simulink model "Inverted_Pendulum9"  (R2020b)
settings: Solver=ode1  StartTime=0.0  StopTime=5  FixedStep=T  RelTol=1e-3  EnableMultiTasking=on
model workspace (MAT data in the model file):
  Var = 0
values from neighbouring files (symbols this model uses):
  binb1 = reshape(psi(binLayerRanges(1, 3):binLayerRanges(1, 4)), binLayers(2), 1)    [main.m]
  binb2 = reshape(psi(binLayerRanges(2, 3):binLayerRanges(2, 4)), binLayers(3), 1)    [main.m]
  binb3 = reshape(psi(binLayerRanges(3, 3):binLayerRanges(3, 4)), binLayers(4), 1)    [main.m]
  binW1 = reshape(psi(binLayerRanges(1, 1):binLayerRanges(1, 2)), binLayers(2), binLayers(1))    [main.m]
  binW2 = reshape(psi(binLayerRanges(2, 1):binLayerRanges(2, 2)), binLayers(3), binLayers(2))    [main.m]
  binW3 = reshape(psi(binLayerRanges(3, 1):binLayerRanges(3, 2)), binLayers(4), binLayers(3))    [main.m]
  control1b1 = reshape(theta1(control1LayerRanges(1, 3):control1LayerRanges(1, 4)), control1Layers(2), 1)    [main.m]
  control1b2 = reshape(theta1(control1LayerRanges(2, 3):control1LayerRanges(2, 4)), control1Layers(3), 1)    [main.m]
  control1b3 = reshape(theta1(control1LayerRanges(3, 3):control1LayerRanges(3, 4)), control1Layers(4), 1)    [main.m]
  control1W1 = reshape(theta1(control1LayerRanges(1, 1):control1LayerRanges(1, 2)), control1Layers(2), control1Layers(1))    [main.m]
  control1W2 = reshape(theta1(control1LayerRanges(2, 1):control1LayerRanges(2, 2)), control1Layers(3), control1Layers(2))    [main.m]
  control1W3 = reshape(theta1(control1LayerRanges(3, 1):control1LayerRanges(3, 2)), control1Layers(4), control1Layers(3))    [main.m]
  control2b1 = reshape(theta2(control2LayerRanges(1, 3):control2LayerRanges(1, 4)), control2Layers(2), 1)    [main.m]
  control2b2 = reshape(theta2(control2LayerRanges(2, 3):control2LayerRanges(2, 4)), control2Layers(3), 1)    [main.m]
  control2b3 = reshape(theta2(control2LayerRanges(3, 3):control2LayerRanges(3, 4)), control2Layers(4), 1)    [main.m]
  control2W1 = reshape(theta2(control2LayerRanges(1, 1):control2LayerRanges(1, 2)), control2Layers(2), control2Layers(1))    [main.m]
  control2W2 = reshape(theta2(control2LayerRanges(2, 1):control2LayerRanges(2, 2)), control2Layers(3), control2Layers(2))    [main.m]
  control2W3 = reshape(theta2(control2LayerRanges(3, 1):control2LayerRanges(3, 2)), control2Layers(4), control2Layers(3))    [main.m]
  control3b1 = reshape(theta3(control3LayerRanges(1, 3):control3LayerRanges(1, 4)), control3Layers(2), 1)    [main.m]
  control3b2 = reshape(theta3(control3LayerRanges(2, 3):control3LayerRanges(2, 4)), control3Layers(3), 1)    [main.m]
  control3b3 = reshape(theta3(control3LayerRanges(3, 3):control3LayerRanges(3, 4)), control3Layers(4), 1)    [main.m]
  control3W1 = reshape(theta3(control3LayerRanges(1, 1):control3LayerRanges(1, 2)), control3Layers(2), control3Layers(1))    [main.m]
  control3W2 = reshape(theta3(control3LayerRanges(2, 1):control3LayerRanges(2, 2)), control3Layers(3), control3Layers(2))    [main.m]
  control3W3 = reshape(theta3(control3LayerRanges(3, 1):control3LayerRanges(3, 2)), control3Layers(4), control3Layers(3))    [main.m]
  g = 9.81    [Inverted_Pendulum9_data.m]
  Jp = m*Lp*Lp/3    (= 0.0056549032375)    [Inverted_Pendulum9_data.m]
  K1 = K(1,1)    [Inverted_Pendulum9_data.m]
  K2 = K(1,2)    [Inverted_Pendulum9_data.m]
  K3 = K(1,3)    [Inverted_Pendulum9_data.m]
  K4 = K(1,4)    [Inverted_Pendulum9_data.m]
  Kenc = 2.275e-5    (= 2.275e-05)    [Inverted_Pendulum9_data.m]    (also in cartpole_data.m = 2.27489350843e-05)
  Kt = 0.00767    [Inverted_Pendulum9_data.m]
  Lp = 0.6413/2    (= 0.32065)    [Inverted_Pendulum9_data.m]
  M = 0.57    [Inverted_Pendulum9_data.m]    (also in cartpole_data.m)
  m = 0.165    [Inverted_Pendulum9_data.m]
  Nenc = 4096    [Inverted_Pendulum9_data.m]    (also in cartpole_data.m)
  R = 2.6    [Inverted_Pendulum9_data.m]    (also in cartpole_data.m)
  rg = 3.71    [Inverted_Pendulum9_data.m]    (also in cartpole_data.m)
  rm = 6.35e-3    (= 0.00635)    [Inverted_Pendulum9_data.m]    (also in cartpole_data.m)
  T = 0.001    [Inverted_Pendulum9_data.m]    (also in cartpole_data.m)
  theta_0 = 1*pi/180    (= 0.0174532925199)    [Inverted_Pendulum9_data.m]
  Vmax = 10    [Inverted_Pendulum9_data.m]
  x_0 = 0*0.1    (= 0)    [Inverted_Pendulum9_data.m]
undefined symbols (not defined in the file or in its folder): af, bf, magnitude
libraries: simulink x1
settings Model: ExtModeArmWhenConnect=off  Creator=johnchiasson  LastModifiedBy=nardosashenafi
settings DataIOCC: LimitDataPoints=on  SaveFormat=Array  SignalLoggingSaveFormat=ModelDataLogs  ReturnWorkspaceOutputs=off
settings OptimizationCC: BooleanDataType=off  OptimizeBlockIOStorage=off  BufferReuse=off  GlobalBufferReuse=off  ExpressionFolding=off  ExpressionDepthLimit=2147483647  LocalBlockOutputs=off  LifeSpan=inf  OptimizeDataStoreBuffers=off  BusAssignmentInplaceUpdate=off
settings DebuggingCC: SaveWithParameterizedLinksMsg=none  UnderspecifiedInitializationDetection=Classic  MergeDetectMultiDrivingBlocksExec=none  SignalResolutionControl=TryResolveAllWithWarning  MultiTaskDSMMsg=warning  MultiTaskCondExecSysMsg=none  FcnCallInpInsideContextMsg=warning  StateNameClashWarn=warning  SFUnexpectedBacktrackingDiag=warning  SFNoUnconditionalDefaultTransitionDiag=warning  SFExecutionAtInitializationDiag=none  UnderSpecifiedDimensionMsg=warning  ArithmeticOperatorsInVariantConditions=warning
settings HardwareCC: ProdBitPerPointer=32  ProdBitPerSizeT=32  ProdBitPerPtrDiffT=32  ProdLargestAtomicFloat=None  ProdIntDivRoundTo=Undefined  ProdEndianess=Unspecified  ProdWordSize=32  ProdHWDeviceType=32-bit Generic  TargetUnknown=on
settings ModelReferenceCC: PropagateSignalLabelsOutOfModel=off
settings SFSimCC: SimUseLocalCustomCode=off  CustomCodeUndefinedFunction=UseInterfaceOnly
settings RTWCC: SystemTargetFile=wincon.tlc  MakeCommand=make_wc  TemplateMakefile=nt_msvc.tmf  RTWUseLocalCustomCode=off
settings CodeAppCC: StateflowObjectComments=on
settings STFCustomTargetCC: ModelReferenceCompliant=off  ConcurrentExecutionCompliant=off  MATLABClassNameForMDSCustomization=Simulink.SoftwareTarget.TargetSpecificTriggerConfigurationBase  CPPClassGenCompliant=off  SystemTargetFile=wincon.tlc
settings ConfigComp: CovMetricSettings=dw  CovSaveCumulativeToWorkspaceVar=on  CovSaveSingleToWorkspaceVar=on  CovExternalEMLEnable=off  CovSFcnEnable=off

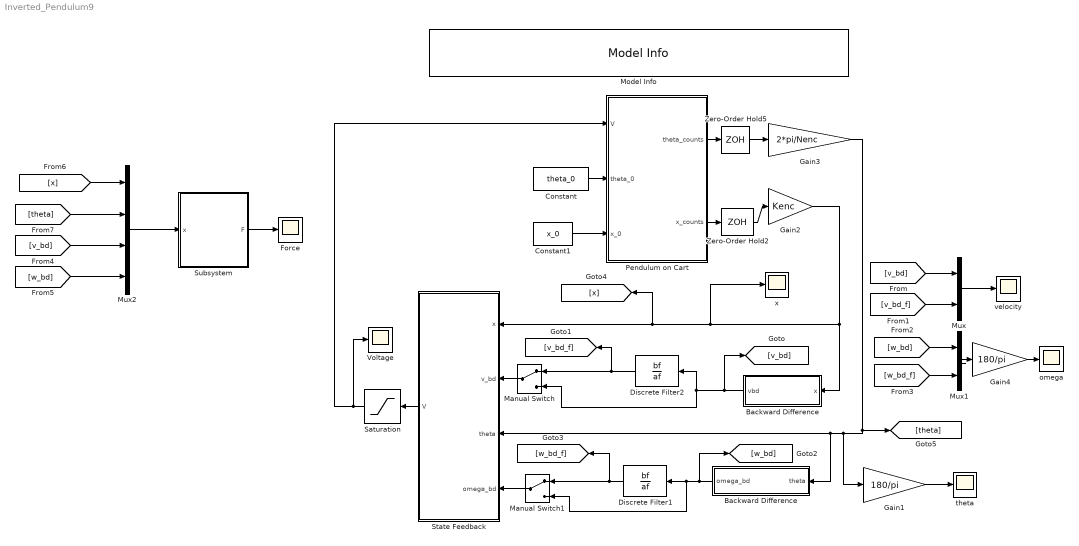
== system Inverted_Pendulum9 ==
  Backward Difference : Subsystem
  "Backward Difference " : Subsystem
  Constant : Constant  Value=theta_0
  Constant1 : Constant  Value=x_0
  Discrete Filter1 : DiscreteFilter  Numerator=bf  Denominator=af
  Discrete Filter2 : DiscreteFilter  Numerator=bf  Denominator=af
  Force : Scope
  Gain1 : Gain  Gain=180/pi  SaturateOnIntegerOverflow=on  OutDataTypeStr=Inherit: Same as input  ParamDataTypeStr=Inherit: Same as input
  Gain2 : Gain  Gain=Kenc  SaturateOnIntegerOverflow=on  OutDataTypeStr=Inherit: Same as input  ParamDataTypeStr=Inherit: Same as input
  Gain3 : Gain  Gain=2*pi/Nenc  SaturateOnIntegerOverflow=on  OutDataTypeStr=Inherit: Same as input  ParamDataTypeStr=Inherit: Same as input
  Gain4 : Gain  Gain=180/pi  SaturateOnIntegerOverflow=on  OutDataTypeStr=Inherit: Same as input  ParamDataTypeStr=Inherit: Same as input
  Manual Switch : ManualSwitch
  Manual Switch1 : ManualSwitch
  Model Info : simulink/Model-Wide Utilities/Model Info  Frame=on  DisplayStringWithTags=Inverted Pendulum on the Cart Model with Encoder Models  HorizontalTextAlignment=Center  LeftAlignmentValue=0.5
  Mux : Mux  Inputs=2
  Mux1 : Mux  Inputs=2
  Mux2 : Mux
  Pendulum on Cart : Subsystem
  Saturation : Saturate  UpperLimit=Vmax  LowerLimit=-Vmax
  State Feedback : Subsystem
  Subsystem : Subsystem
  Voltage : Scope
  Zero-Order Hold2 : ZeroOrderHold  SampleTime=T
  Zero-Order Hold5 : ZeroOrderHold  SampleTime=T
  omega : Scope
  theta : Scope
  velocity : Scope
  x : Scope
  wires:
  State Feedback/1(V) -> Saturation/1
  Constant/1 -> Pendulum on Cart/2(theta_0)
  Constant1/1 -> Pendulum on Cart/3(x_0)
  "Backward Difference "/1(vbd) -> Manual Switch/2, Discrete Filter2/1, [v_bd]
  Pendulum on Cart/2(x_counts) -> Zero-Order Hold2/1
  Pendulum on Cart/1(theta_counts) -> Zero-Order Hold5/1
  Saturation/1 -> Pendulum on Cart/1(V), Voltage/1
  Mux/1 -> velocity/1
  [v_bd] -> Mux/1
  [v_bd_f] -> Mux/2
  Backward Difference/1(omega_bd) -> [w_bd], Manual Switch1/2, Discrete Filter1/1
  Mux1/1 -> Gain4/1
  [w_bd] -> Mux1/1
  [w_bd_f] -> Mux1/2
  Gain1/1 -> theta/1
  Gain4/1 -> omega/1
  Gain3/1 -> Gain1/1, State Feedback/3(theta), Backward Difference/1(theta), [theta]
  Gain2/1 -> [x], State Feedback/1(x), x/1, "Backward Difference "/1(x)
  Zero-Order Hold5/1 -> Gain3/1
  Zero-Order Hold2/1 -> Gain2/1
  Discrete Filter2/1 -> Manual Switch/1, [v_bd_f]
  Discrete Filter1/1 -> [w_bd_f], Manual Switch1/1
  Manual Switch/1 -> State Feedback/2(v_bd)
  Manual Switch1/1 -> State Feedback/4(omega_bd)
  [w_bd] -> Mux2/4
  [v_bd] -> Mux2/3
  [theta] -> Mux2/2
  [x] -> Mux2/1
  Mux2/1 -> Subsystem/1(x)
  Subsystem/1(F) -> Force/1

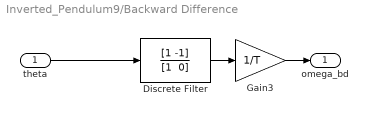
== system Inverted_Pendulum9/Backward Difference ==
  theta : Inport
  Discrete Filter : DiscreteFilter  Numerator=[1 -1]  Denominator="[1  0]"
  Gain3 : Gain  Gain=1/T  SaturateOnIntegerOverflow=on  OutDataTypeStr=Inherit: Same as input  ParamDataTypeStr=Inherit: Same as input
  omega_bd : Outport  VectorParamsAs1DForOutWhenUnconnected=off
  wires:
  Discrete Filter/1 -> Gain3/1
  Gain3/1 -> omega_bd/1
  theta/1 -> Discrete Filter/1

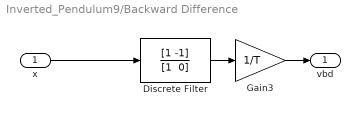
== system Inverted_Pendulum9/Backward Difference  ==
  x : Inport
  Discrete Filter : DiscreteFilter  Numerator=[1 -1]  Denominator="[1  0]"
  Gain3 : Gain  Gain=1/T  SaturateOnIntegerOverflow=on  OutDataTypeStr=Inherit: Same as input  ParamDataTypeStr=Inherit: Same as input
  vbd : Outport  VectorParamsAs1DForOutWhenUnconnected=off
  wires:
  Discrete Filter/1 -> Gain3/1
  Gain3/1 -> vbd/1
  x/1 -> Discrete Filter/1

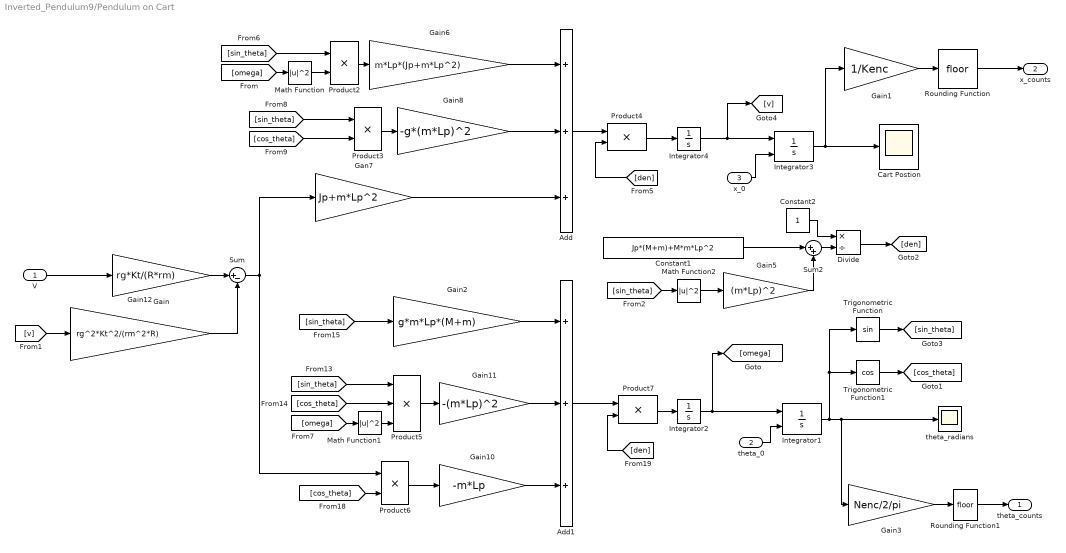
== system Inverted_Pendulum9/Pendulum on Cart ==
  V : Inport
  theta_0 : Inport  Port=2
  x_0 : Inport  Port=3
  Add : Sum  Inputs=+++
  Add1 : Sum  Inputs=+++
  Cart Postion : Scope
  Constant1 : Constant  Value=Jp*(M+m)+M*m*Lp^2
  Constant2 : Constant
  Divide : Product  Inputs=*/
  Gain : Gain  Gain=rg*Kt/(R*rm)  SaturateOnIntegerOverflow=on  OutDataTypeStr=Inherit: Same as input  ParamDataTypeStr=Inherit: Same as input
  Gain1 : Gain  Gain=1/Kenc  SaturateOnIntegerOverflow=on  OutDataTypeStr=Inherit: Same as input  ParamDataTypeStr=Inherit: Same as input
  Gain10 : Gain  Gain=-m*Lp  SaturateOnIntegerOverflow=on  OutDataTypeStr=Inherit: Same as input  ParamDataTypeStr=Inherit: Same as input
  Gain11 : Gain  Gain=-(m*Lp)^2  SaturateOnIntegerOverflow=on  OutDataTypeStr=Inherit: Same as input  ParamDataTypeStr=Inherit: Same as input
  Gain12 : Gain  Gain=rg^2*Kt^2/(rm^2*R)  SaturateOnIntegerOverflow=on  OutDataTypeStr=Inherit: Same as input  ParamDataTypeStr=Inherit: Same as input
  Gain2 : Gain  Gain=g*m*Lp*(M+m)  SaturateOnIntegerOverflow=on  OutDataTypeStr=Inherit: Same as input  ParamDataTypeStr=Inherit: Same as input
  Gain3 : Gain  Gain=Nenc/2/pi  SaturateOnIntegerOverflow=on  OutDataTypeStr=Inherit: Same as input  ParamDataTypeStr=Inherit: Same as input
  Gain5 : Gain  Gain=(m*Lp)^2  SaturateOnIntegerOverflow=on  OutDataTypeStr=Inherit: Same as input  ParamDataTypeStr=Inherit: Same as input
  Gain6 : Gain  Gain=m*Lp*(Jp+m*Lp^2)  SaturateOnIntegerOverflow=on  OutDataTypeStr=Inherit: Same as input  ParamDataTypeStr=Inherit: Same as input
  Gain8 : Gain  Gain=-g*(m*Lp)^2  SaturateOnIntegerOverflow=on  OutDataTypeStr=Inherit: Same as input  ParamDataTypeStr=Inherit: Same as input
  Gan7 : Gain  Gain=Jp+m*Lp^2  SaturateOnIntegerOverflow=on  OutDataTypeStr=Inherit: Same as input  ParamDataTypeStr=Inherit: Same as input
  Integrator1 : Integrator  InitialConditionSource=external  InitialCondition=0.3
  Integrator2 : Integrator
  Integrator3 : Integrator  InitialConditionSource=external
  Integrator4 : Integrator
  Math Function : Math  Operator=magnitude^2  SignedPower=on  SaturateOnIntegerOverflow=on
  Math Function1 : Math  Operator=magnitude^2  SignedPower=on  SaturateOnIntegerOverflow=on
  Math Function2 : Math  Operator=magnitude^2  SignedPower=on  SaturateOnIntegerOverflow=on
  Product{2..4,6..7} (5 alike) : Product  InputSameDT=on  RndMeth=Zero  SaturateOnIntegerOverflow=on  OutDataTypeStr=Inherit: Same as first input
  Product5 : Product  Inputs=3  InputSameDT=on  RndMeth=Zero  SaturateOnIntegerOverflow=on  OutDataTypeStr=Inherit: Same as first input
  Rounding Function : Rounding
  Rounding Function1 : Rounding
  Sum : Sum  Inputs=|+-  InputSameDT=on  SaturateOnIntegerOverflow=on  OutDataTypeStr=Inherit: Same as first input
  Sum2 : Sum  Inputs=|++
  Trigonometric Function : Trigonometry
  Trigonometric Function1 : Trigonometry  Operator=cos
  theta_radians : Scope
  theta_counts : Outport  VectorParamsAs1DForOutWhenUnconnected=off
  x_counts : Outport  Port=2  VectorParamsAs1DForOutWhenUnconnected=off
  wires:
  Integrator2/1 -> [omega], Integrator1/1
  Integrator1/1 -> Trigonometric Function1/1, Trigonometric Function/1, theta_radians/1, Gain3/1
  Integrator4/1 -> [v], Integrator3/1
  Integrator3/1 -> Cart Postion/1, Gain1/1
  theta_0/1 -> Integrator1/2
  x_0/1 -> Integrator3/2
  [sin_theta] -> Math Function2/1
  Constant1/1 -> Sum2/1
  Gain5/1 -> Sum2/2
  Sum2/1 -> Divide/2
  Constant2/1 -> Divide/1
  Divide/1 -> [den]
  Trigonometric Function/1 -> [sin_theta]
  Trigonometric Function1/1 -> [cos_theta]
  Math Function/1 -> Product2/2
  [omega] -> Math Function/1
  [sin_theta] -> Product2/1
  Product2/1 -> Gain6/1
  [cos_theta] -> Product3/2
  [sin_theta] -> Product3/1
  Product3/1 -> Gain8/1
  Add/1 -> Product4/1
  [den] -> Product4/2
  Product4/1 -> Integrator4/1
  [sin_theta] -> Gain2/1
  [cos_theta] -> Product5/2
  [sin_theta] -> Product5/1
  Product5/1 -> Gain11/1
  Math Function1/1 -> Product5/3
  [omega] -> Math Function1/1
  [cos_theta] -> Product6/2
  Product6/1 -> Gain10/1
  [den] -> Product7/2
  Add1/1 -> Product7/1
  Product7/1 -> Integrator2/1
  Gain1/1 -> Rounding Function/1
  Rounding Function/1 -> x_counts/1
  Gain3/1 -> Rounding Function1/1
  Rounding Function1/1 -> theta_counts/1
  V/1 -> Gain/1
  Sum/1 -> Product6/1, Gan7/1
  Math Function2/1 -> Gain5/1
  Gain6/1 -> Add/1
  Gan7/1 -> Add/3
  Gain2/1 -> Add1/1
  Gain11/1 -> Add1/2
  Gain10/1 -> Add1/3
  Gain8/1 -> Add/2
  Gain/1 -> Sum/1
  Gain12/1 -> Sum/2
  [v] -> Gain12/1

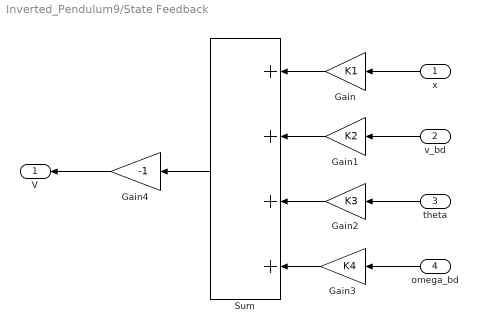
== system Inverted_Pendulum9/State Feedback ==
  x : Inport
  v_bd : Inport  Port=2
  theta : Inport  Port=3
  omega_bd : Inport  Port=4
  Gain : Gain  Gain=K1  SaturateOnIntegerOverflow=on  OutDataTypeStr=Inherit: Same as input  ParamDataTypeStr=Inherit: Same as input
  Gain1 : Gain  Gain=K2  SaturateOnIntegerOverflow=on  OutDataTypeStr=Inherit: Same as input  ParamDataTypeStr=Inherit: Same as input
  Gain2 : Gain  Gain=K3  SaturateOnIntegerOverflow=on  OutDataTypeStr=Inherit: Same as input  ParamDataTypeStr=Inherit: Same as input
  Gain3 : Gain  Gain=K4  SaturateOnIntegerOverflow=on  OutDataTypeStr=Inherit: Same as input  ParamDataTypeStr=Inherit: Same as input
  Gain4 : Gain  Gain=-1  SaturateOnIntegerOverflow=on  OutDataTypeStr=Inherit: Same as input  ParamDataTypeStr=Inherit: Same as input
  Sum : Sum  Inputs=++++  InputSameDT=on  SaturateOnIntegerOverflow=on  OutDataTypeStr=Inherit: Same as first input
  V : Outport  VectorParamsAs1DForOutWhenUnconnected=off
  wires:
  Gain/1 -> Sum/1
  Gain1/1 -> Sum/2
  Gain2/1 -> Sum/3
  Gain3/1 -> Sum/4
  omega_bd/1 -> Gain3/1
  theta/1 -> Gain2/1
  v_bd/1 -> Gain1/1
  x/1 -> Gain/1
  Sum/1 -> Gain4/1
  Gain4/1 -> V/1

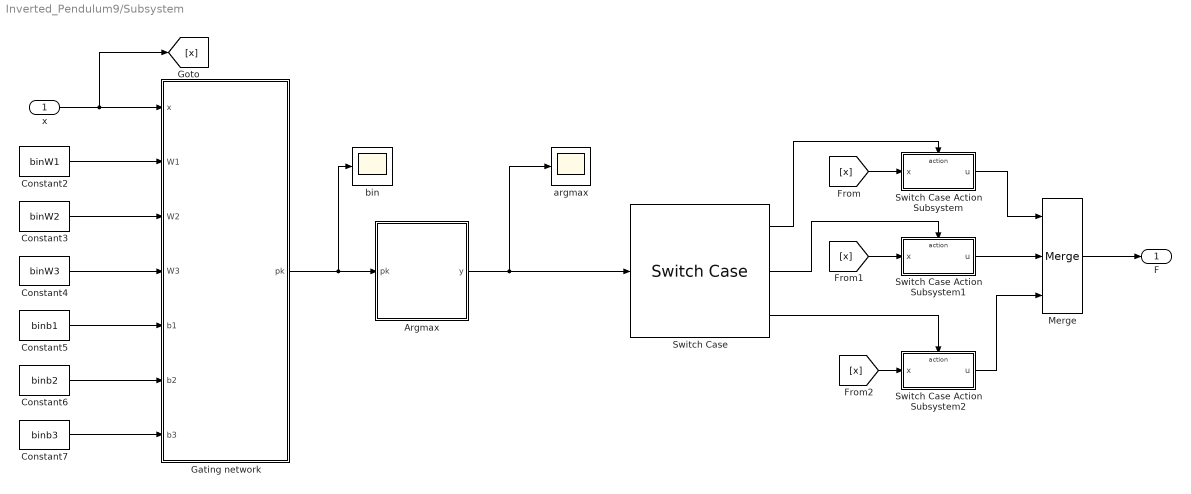
== system Inverted_Pendulum9/Subsystem ==
  x : Inport
  Argmax : MATLAB Function  TreatAsAtomicUnit=on
  Constant2 : Constant  Value=binW1
  Constant3 : Constant  Value=binW2
  Constant4 : Constant  Value=binW3
  Constant5 : Constant  Value=binb1
  Constant6 : Constant  Value=binb2
  Constant7 : Constant  Value=binb3
  Gating network : MATLAB Function  TreatAsAtomicUnit=on
  Merge : Merge  Inputs=3
  Switch Case : SwitchCase  CaseConditions={1, 2, 3}  ShowDefaultCase=off
  Switch Case Action Subsystem : Subsystem  TreatAsAtomicUnit=on
  Switch Case Action Subsystem1 : Subsystem  TreatAsAtomicUnit=on
  Switch Case Action Subsystem2 : Subsystem  TreatAsAtomicUnit=on
  argmax : Scope
  bin : Scope
  F : Outport  VectorParamsAs1DForOutWhenUnconnected=off
  wires:
  Constant3/1 -> Gating network/3(W2)
  Constant7/1 -> Gating network/7(b3)
  Constant5/1 -> Gating network/5(b1)
  Constant4/1 -> Gating network/4(W3)
  Constant6/1 -> Gating network/6(b2)
  Gating network/1(pk) -> Argmax/1(pk), bin/1
  Constant2/1 -> Gating network/2(W1)
  x/1 -> [x], Gating network/1(x)
  Argmax/1(y) -> argmax/1, Switch Case/1
  Switch Case/1 -> Switch Case Action Subsystem/Action
  Switch Case/2 -> Switch Case Action Subsystem1/Action
  Switch Case/3 -> Switch Case Action Subsystem2/Action
  [x] -> Switch Case Action Subsystem2/1(x)
  [x] -> Switch Case Action Subsystem1/1(x)
  [x] -> Switch Case Action Subsystem/1(x)
  Switch Case Action Subsystem/1(u) -> Merge/1
  Switch Case Action Subsystem1/1(u) -> Merge/2
  Switch Case Action Subsystem2/1(u) -> Merge/3
  Merge/1 -> F/1

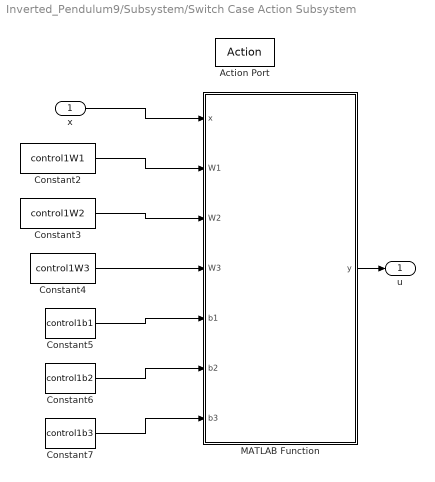
== system Inverted_Pendulum9/Subsystem/Switch Case Action Subsystem ==
  x : Inport
  Action Port : ActionPort  ActionPortLabel=case [ 1 ]:
  Constant2 : Constant  Value=control1W1
  Constant3 : Constant  Value=control1W2
  Constant4 : Constant  Value=control1W3  VectorParams1D=off
  Constant5 : Constant  Value=control1b1
  Constant6 : Constant  Value=control1b2
  Constant7 : Constant  Value=control1b3
  MATLAB Function : MATLAB Function  TreatAsAtomicUnit=on
  u : Outport
  wires:
  Constant2/1 -> MATLAB Function/2(W1)
  Constant5/1 -> MATLAB Function/5(b1)
  Constant7/1 -> MATLAB Function/7(b3)
  Constant6/1 -> MATLAB Function/6(b2)
  Constant4/1 -> MATLAB Function/4(W3)
  Constant3/1 -> MATLAB Function/3(W2)
  x/1 -> MATLAB Function/1(x)
  MATLAB Function/1(y) -> u/1

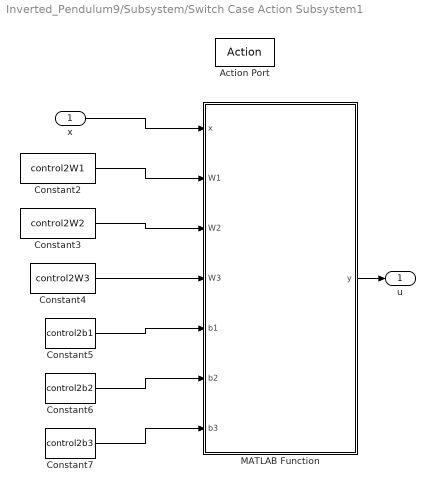
== system Inverted_Pendulum9/Subsystem/Switch Case Action Subsystem1 ==
  x : Inport
  Action Port : ActionPort  ActionPortLabel=case [ 2 ]:
  Constant2 : Constant  Value=control2W1
  Constant3 : Constant  Value=control2W2
  Constant4 : Constant  Value=control2W3  VectorParams1D=off
  Constant5 : Constant  Value=control2b1
  Constant6 : Constant  Value=control2b2
  Constant7 : Constant  Value=control2b3
  MATLAB Function : MATLAB Function  TreatAsAtomicUnit=on
  u : Outport
  wires:
  Constant7/1 -> MATLAB Function/7(b3)
  Constant2/1 -> MATLAB Function/2(W1)
  Constant3/1 -> MATLAB Function/3(W2)
  Constant4/1 -> MATLAB Function/4(W3)
  MATLAB Function/1(y) -> u/1
  x/1 -> MATLAB Function/1(x)
  Constant6/1 -> MATLAB Function/6(b2)
  Constant5/1 -> MATLAB Function/5(b1)

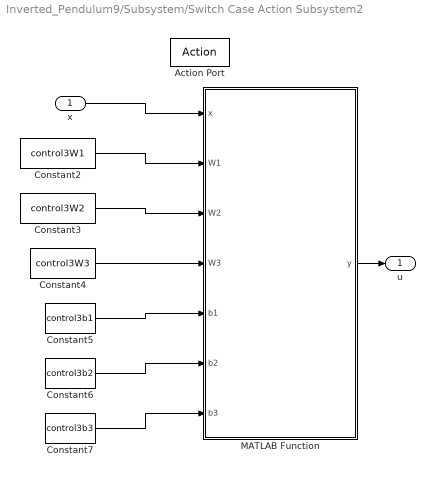
== system Inverted_Pendulum9/Subsystem/Switch Case Action Subsystem2 ==
  x : Inport
  Action Port : ActionPort  ActionPortLabel=case [ 3 ]:
  Constant2 : Constant  Value=control3W1
  Constant3 : Constant  Value=control3W2
  Constant4 : Constant  Value=control3W3  VectorParams1D=off
  Constant5 : Constant  Value=control3b1
  Constant6 : Constant  Value=control3b2
  Constant7 : Constant  Value=control3b3
  MATLAB Function : MATLAB Function  TreatAsAtomicUnit=on
  u : Outport
  wires:
  Constant7/1 -> MATLAB Function/7(b3)
  Constant2/1 -> MATLAB Function/2(W1)
  Constant3/1 -> MATLAB Function/3(W2)
  Constant4/1 -> MATLAB Function/4(W3)
  MATLAB Function/1(y) -> u/1
  x/1 -> MATLAB Function/1(x)
  Constant6/1 -> MATLAB Function/6(b2)
  Constant5/1 -> MATLAB Function/5(b1)

== matlab function Inverted_Pendulum9/Subsystem/Argmax ==
  data: pk input; y output
function y = fcn(pk)
    maxindex = 1;
    for i = 1:length(pk)-1
       if pk(i+1) > pk(maxindex)
           maxindex = i+1;
       end
    end
y = maxindex;

== matlab function Inverted_Pendulum9/Subsystem/Gating network ==
  data: x input; W1 input; pk output; W2 input; W3 input; b1 input; b2 input; b3 input
function pk = fcn(x, W1, W2, W3, b1, b2, b3)

    z0 = [x(1); cos(x(2)); sin(x(2)); x(3); x(4)];
    z1 = elu(W1*z0 + b1);
    z2 = elu(W2*z1 + b2);
    z3 = W3*z2 + b3;
    pk = softmax(z3);
    
end
    
function y = softmax(x)
    y = zeros(length(x));
    for i =1:length(x)
        y(i) = exp(x(i))/sum(exp(x));
    end
end

== matlab function Inverted_Pendulum9/Subsystem/Switch Case Action Subsystem/MATLAB Function ==
  data: x input; y output; W1 input; W2 input; W3 input; b1 input; b2 input; b3 input
function y = fcn(x, W1, W2, W3, b1, b2, b3)
    z0 = [x(1); cos(x(2)); sin(x(2)); x(3); x(4)];
    z1 = elu(W1*z0 + b1);
    z2 = elu(W2*z1 + b2);
    z3 = W3*z2 + b3;
y = z3;

== matlab function Inverted_Pendulum9/Subsystem/Switch Case Action Subsystem1/MATLAB Function ==
  data: x input; y output; W1 input; W2 input; W3 input; b1 input; b2 input; b3 input
function y = fcn(x, W1, W2, W3, b1, b2, b3)
    z0 = [x(1); cos(x(2)); sin(x(2)); x(3); x(4)];
    z1 = elu(W1*z0 + b1);
    z2 = elu(W2*z1 + b2);
    z3 = W3*z2 + b3;
y = z3;

== matlab function Inverted_Pendulum9/Subsystem/Switch Case Action Subsystem2/MATLAB Function ==
  data: x input; y output; W1 input; W2 input; W3 input; b1 input; b2 input; b3 input
function y = fcn(x, W1, W2, W3, b1, b2, b3)
    z0 = [x(1); cos(x(2)); sin(x(2)); x(3); x(4)];
    z1 = elu(W1*z0 + b1);
    z2 = elu(W2*z1 + b2);
    z3 = W3*z2 + b3;
y = z3;
